simulink model "Modello_Irb1300_controllo_dinamico"  (R2024a)
settings: Solver=FixedStepAuto  StartTime=0.0  StopTime=16.0  FixedStep=0.05  RelTol=1e-3
values from neighbouring files (symbols this model uses):
  DH = [ ... (first row only)    [BackupRUN1.m]    (also in BackupRUN2.m; IRB1300_ABB6DOF_bodytree_mesh_RUN2.m)
undefined symbols (not defined in the file or in its folder): DiscIntNeverNeededParam, rb
libraries: vrlib x1
settings Model: Creator=giaki  LastModifiedBy=giaki
settings DataIOCC: SignalLogging=off

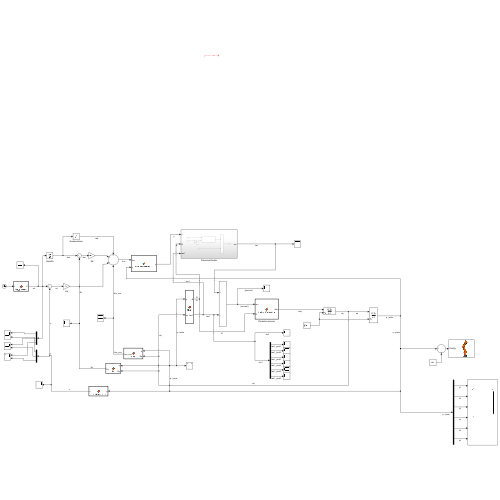
[thumbnail: Simulink's stored preview of the top-level diagram]
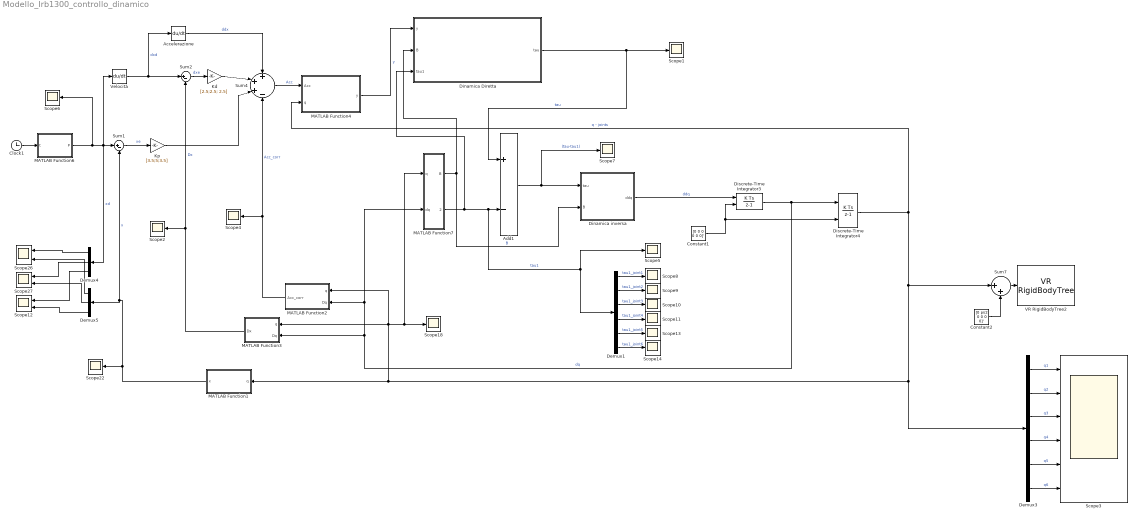
== system Modello_Irb1300_controllo_dinamico ==
  Accelerazione : Derivative
  Add1 : Sum  Inputs=+-
  Clock1 : Clock
  Constant1 : Constant  Value=[0 0 0 0 0 0]'
  Constant2 : Constant  Value=[0 pi/2 0 0 0 0]'
  Demux1 : Demux  Outputs=6
  Demux3 : Demux  Outputs=6
  Demux4 : Demux  Outputs=3
  Demux5 : Demux  Outputs=3
  Dinamica Diretta : Subsystem
  Dinamica inversa : MATLAB Function  TreatAsAtomicUnit=on
  Discrete-Time Integrator3 : DiscreteIntegrator  InitialConditionSource=external  SampleTime=-1  ICPrevOutput=DiscIntNeverNeededParam  ICPrevScaledInput=DiscIntNeverNeededParam
  Discrete-Time Integrator4 : DiscreteIntegrator  InitialConditionSource=external  SampleTime=-1  ICPrevOutput=DiscIntNeverNeededParam  ICPrevScaledInput=DiscIntNeverNeededParam
  Kd : Gain  Gain=[2.5;2.5; 2.5]
  Kp : Gain  Gain=[3.5;5;3.5]
  MATLAB Function1 : MATLAB Function  TreatAsAtomicUnit=on
  MATLAB Function2 : MATLAB Function  TreatAsAtomicUnit=on
  MATLAB Function3 : MATLAB Function  TreatAsAtomicUnit=on
  MATLAB Function4 : MATLAB Function  TreatAsAtomicUnit=on
  MATLAB Function6 : MATLAB Function  TreatAsAtomicUnit=on
  MATLAB Function7 : MATLAB Function  TreatAsAtomicUnit=on
  Scope{1..2,4..11,13..14,18,22} (14 alike) : Scope
  Scope12 : Scope  NumInputPorts=2
  Scope26 : Scope  NumInputPorts=2
  Scope27 : Scope  NumInputPorts=2
  Scope3 : Scope  NumInputPorts=6
  Sum1 : Sum  Inputs=|+-
  Sum2 : Sum  Inputs=|+-
  Sum4 : Sum  Inputs=+++-
  Sum7 : Sum  Inputs=|++
  VR RigidBodyTree2 : vrlib/VR RigidBodyTree  VrmlFile=robot_scene_2.x3d  RBT=Irb1300  useRBT=on  Ts=0.1  ForceViewerOpen=on
  Velocità : Derivative
  wires:
  ? -> ?
  MATLAB Function6/1(P) -> Scope6/1, Demux4/1, Sum1/1, Velocità/1  "xd"
  Demux4/2 -> Scope27/1
  Clock1/1 -> MATLAB Function6/1(t)
  Discrete-Time Integrator4/1 -> MATLAB Function1/1(q), MATLAB Function2/1(q), MATLAB Function3/1(q), Scope18/1, MATLAB Function7/1(q), Demux3/1, Sum7/1, MATLAB Function4/2(q)  "q - joints"
  MATLAB Function1/1(x) -> Sum1/2, Demux5/1, Scope22/1  "x"
  Sum2/1 -> Kd/1  "dxe"
  Demux4/3 -> Scope12/1
  MATLAB Function3/1(Dx) -> Scope2/1, Sum2/2  "Dx"
  Demux3/1 -> Scope3/1  "q1"
  Sum4/1 -> MATLAB Function4/1(Acc)  "Acc"
  Kd/1 -> Sum4/2
  Constant1/1 -> Discrete-Time Integrator3/2, Discrete-Time Integrator4/2
  Accelerazione/1 -> Sum4/1  "ddx"
  Demux5/1 -> Scope26/2
  Dinamica inversa/1(ddq) -> Discrete-Time Integrator3/1  "ddq"
  Demux3/3 -> Scope3/3  "q3"
  Add1/1 -> Scope7/1, Dinamica inversa/1(tau)  "(tau-tau1)"
  Discrete-Time Integrator3/1 -> MATLAB Function3/2(Dq), MATLAB Function7/2(dq), MATLAB Function2/2(Dq), Discrete-Time Integrator4/1  "dq"
  Sum1/1 -> Kp/1  "xe"
  Velocità/1 -> Sum2/1, Accelerazione/1  "dxd"
  MATLAB Function7/1(B) -> Dinamica Diretta/2(B), Dinamica inversa/2(B)  "B"
  Demux5/2 -> Scope27/2
  Dinamica Diretta/1(tau) -> Scope1/1, Add1/1  "tau"
  Demux3/5 -> Scope3/5  "q5"
  Sum7/1 -> VR RigidBodyTree2/1
  Demux4/1 -> Scope26/1
  Demux3/6 -> Scope3/6  "q6"
  Demux3/4 -> Scope3/4  "q4"
  Demux5/3 -> Scope12/2
  Constant2/1 -> Sum7/2
  MATLAB Function2/1(Acc_corr) -> Scope4/1, Sum4/4  "Acc_corr"
  MATLAB Function4/1(y) -> Dinamica Diretta/1(y)  "y"
  Demux3/2 -> Scope3/2  "q2"
  Kp/1 -> Sum4/3
  MATLAB Function7/2(tau1) -> Demux1/1, Scope5/1, Add1/2, Dinamica Diretta/3(tau1)  "tau1"
  Demux1/1 -> Scope8/1  "tau1_joint1"
  Demux1/2 -> Scope9/1  "tau1_joint2"
  Demux1/3 -> Scope10/1  "tau1_joint3"
  Demux1/4 -> Scope11/1  "tau1_joint4"
  Demux1/5 -> Scope13/1  "tau1_joint5"
  Demux1/6 -> Scope14/1  "tau1_joint6"

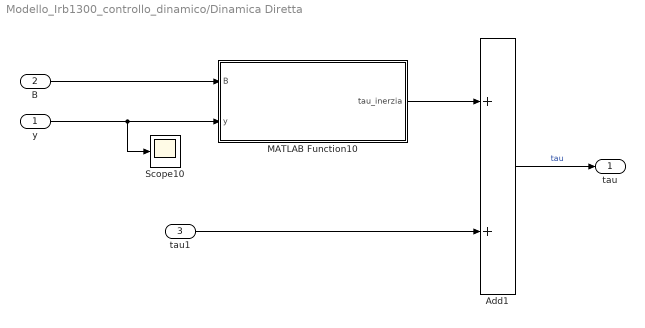
== system Modello_Irb1300_controllo_dinamico/Dinamica Diretta ==
  y : Inport
  B : Inport  Port=2
  tau1 : Inport  Port=3
  Add1 : Sum
  MATLAB Function10 : MATLAB Function  TreatAsAtomicUnit=on
  Scope10 : Scope
  tau : Outport
  wires:
  B/1 -> MATLAB Function10/1(B)
  MATLAB Function10/1(tau_inerzia) -> Add1/1
  y/1 -> Scope10/1, MATLAB Function10/2(y)
  Add1/1 -> tau/1  "tau"
  tau1/1 -> Add1/2

== matlab function Modello_Irb1300_controllo_dinamico/Dinamica Diretta/MATLAB Function10 ==
  data: B input size=[6,6]; tau_inerzia output; y input size=[6,1]
function tau_inerzia = calcolaTauInerzia(B,y)
    tau_inerzia = B*y;
end

== matlab function Modello_Irb1300_controllo_dinamico/MATLAB Function1 ==
  data: q input; x output
function x = directKinematics(q)

th1 = q(1);
th2 = q(2);
th3 = q(3);
th4 = q(4);
th5 = q(5);
th6 = q(6);

% T06

T = [
[  sin(th6)*(cos(th4)*sin(th1) + sin(th4)*(cos(th1)*sin(th3)*sin(th2 + pi/2) - cos(th1)*cos(th3)*cos(th2 + pi/2))) + cos(th6)*(cos(th5)*(sin(th1)*sin(th4) - cos(th4)*(cos(th1)*sin(th3)*sin(th2 + pi/2) - cos(th1)*cos(th3)*cos(th2 + pi/2))) - sin(th5)*(cos(th1)*cos(th3)*sin(th2 + pi/2) + cos(th1)*cos(th2 + pi/2)*sin(th3))), cos(th6)*(cos(th4)*sin(th1) + sin(th4)*(cos(th1)*sin(th3)*sin(th2 + pi/2) - cos(th1)*cos(th3)*cos(th2 + pi/2))) - sin(th6)*(cos(th5)*(sin(th1)*sin(th4) - cos(th4)*(cos(th1)*sin(th3)*sin(th2 + pi/2) - cos(th1)*cos(th3)*cos(th2 + pi/2))) - sin(th5)*(cos(th1)*cos(th3)*sin(th2 + pi/2) + cos(th1)*cos(th2 + pi/2)*sin(th3))), sin(th5)*(sin(th1)*sin(th4) - cos(th4)*(cos(th1)*sin(th3)*sin(th2 + pi/2) - cos(th1)*cos(th3)*cos(th2 + pi/2))) + cos(th5)*(cos(th1)*cos(th3)*sin(th2 + pi/2) + cos(th1)*cos(th2 + pi/2)*sin(th3)), cos(th1)/20 + (17*cos(th1)*cos(th2 + pi/2))/40 + (9*sin(th5)*(sin(th1)*sin(th4) - cos(th4)*(cos(th1)*sin(th3)*sin(th2 + pi/2) - cos(th1)*cos(th3)*cos(th2 + pi/2))))/50 + (9*cos(th5)*(cos(th1)*cos(th3)*sin(th2 + pi/2) + cos(th1)*cos(th2 + pi/2)*sin(th3)))/50 + (17*cos(th1)*cos(th3)*sin(th2 + pi/2))/40 + (17*cos(th1)*cos(th2 + pi/2)*sin(th3))/40 - (cos(th1)*sin(th3)*sin(th2 + pi/2))/25 + (cos(th1)*cos(th3)*cos(th2 + pi/2))/25]
[- sin(th6)*(cos(th1)*cos(th4) + sin(th4)*(cos(th3)*cos(th2 + pi/2)*sin(th1) - sin(th1)*sin(th3)*sin(th2 + pi/2))) - cos(th6)*(cos(th5)*(cos(th1)*sin(th4) - cos(th4)*(cos(th3)*cos(th2 + pi/2)*sin(th1) - sin(th1)*sin(th3)*sin(th2 + pi/2))) + sin(th5)*(cos(th3)*sin(th1)*sin(th2 + pi/2) + cos(th2 + pi/2)*sin(th1)*sin(th3))), sin(th6)*(cos(th5)*(cos(th1)*sin(th4) - cos(th4)*(cos(th3)*cos(th2 + pi/2)*sin(th1) - sin(th1)*sin(th3)*sin(th2 + pi/2))) + sin(th5)*(cos(th3)*sin(th1)*sin(th2 + pi/2) + cos(th2 + pi/2)*sin(th1)*sin(th3))) - cos(th6)*(cos(th1)*cos(th4) + sin(th4)*(cos(th3)*cos(th2 + pi/2)*sin(th1) - sin(th1)*sin(th3)*sin(th2 + pi/2))), cos(th5)*(cos(th3)*sin(th1)*sin(th2 + pi/2) + cos(th2 + pi/2)*sin(th1)*sin(th3)) - sin(th5)*(cos(th1)*sin(th4) - cos(th4)*(cos(th3)*cos(th2 + pi/2)*sin(th1) - sin(th1)*sin(th3)*sin(th2 + pi/2))), sin(th1)/20 + (17*cos(th2 + pi/2)*sin(th1))/40 - (9*sin(th5)*(cos(th1)*sin(th4) - cos(th4)*(cos(th3)*cos(th2 + pi/2)*sin(th1) - sin(th1)*sin(th3)*sin(th2 + pi/2))))/50 + (9*cos(th5)*(cos(th3)*sin(th1)*sin(th2 + pi/2) + cos(th2 + pi/2)*sin(th1)*sin(th3)))/50 + (cos(th3)*cos(th2 + pi/2)*sin(th1))/25 + (17*cos(th3)*sin(th1)*sin(th2 + pi/2))/40 + (17*cos(th2 + pi/2)*sin(th1)*sin(th3))/40 - (sin(th1)*sin(th3)*sin(th2 + pi/2))/25]
[                                                                                                    cos(th6)*(sin(th5)*(cos(th3)*cos(th2 + pi/2) - sin(th3)*sin(th2 + pi/2)) + cos(th4)*cos(th5)*(cos(th3)*sin(th2 + pi/2) + cos(th2 + pi/2)*sin(th3))) - sin(th4)*sin(th6)*(cos(th3)*sin(th2 + pi/2) + cos(th2 + pi/2)*sin(th3)),                                                                                                 - sin(th6)*(sin(th5)*(cos(th3)*cos(th2 + pi/2) - sin(th3)*sin(th2 + pi/2)) + cos(th4)*cos(th5)*(cos(th3)*sin(th2 + pi/2) + cos(th2 + pi/2)*sin(th3))) - cos(th6)*sin(th4)*(cos(th3)*sin(th2 + pi/2) + cos(th2 + pi/2)*sin(th3)),                                                           cos(th4)*sin(th5)*(cos(th3)*sin(th2 + pi/2) + cos(th2 + pi/2)*sin(th3)) - cos(th5)*(cos(th3)*cos(th2 + pi/2) - sin(th3)*sin(th2 + pi/2)),                                                                                                             (17*sin(th2 + pi/2))/40 - (17*cos(th3)*cos(th2 + pi/2))/40 + (cos(th3)*sin(th2 + pi/2))/25 + (cos(th2 + pi/2)*sin(th3))/25 + (17*sin(th3)*sin(th2 + pi/2))/40 - (9*cos(th5)*(cos(th3)*cos(th2 + pi/2) - sin(th3)*sin(th2 + pi/2)))/50 + (9*cos(th4)*sin(th5)*(cos(th3)*sin(th2 + pi/2) + cos(th2 + pi/2)*sin(th3)))/50 + 68/125]
[                                                                                                                                                                                                                                                                                                                                0,                                                                                                                                                                                                                                                                                                                               0,                                                                                                                                                                                                  0,                                                                                                                                                                                                                                                                                                                                                                                                                                           1]
 ];

x = T(1:3,4); % si estraggono i primi 3 valori della 4 colonna della T06 che rappresentano il vettore delle traslazioni 

end

== matlab function Modello_Irb1300_controllo_dinamico/MATLAB Function2 ==
  data: q input; Acc_corr output; Dq input
function Acc_corr = DJa(q,Dq)

th1 = q(1);
th2 = q(2);
th3 = q(3);
th4 = q(4);
th5 = q(5);
th6 = q(6);

% Velocità di giunto 
dth1 = Dq(1);
dth2 = Dq(2);
dth3 = Dq(3);
dth4 = Dq(4);
dth5 = Dq(5);
dth6 = Dq(6);


% Per il calcolo del DJ viene utilizzato lo script
% JacobianDerive_wrt_time.m 
% Viene utilizzato il DJ = DJp [3X1] di posizione


DJ = [
[(9*sin(th5)*(cos(th4)*(dth1*cos(th1)*sin(th3)*sin(th2 + pi/2) - dth1*cos(th1)*cos(th3)*cos(th2 + pi/2) + dth2*cos(th3)*sin(th1)*sin(th2 + pi/2) + dth2*cos(th2 + pi/2)*sin(th1)*sin(th3) + dth3*cos(th3)*sin(th1)*sin(th2 + pi/2) + dth3*cos(th2 + pi/2)*sin(th1)*sin(th3)) + dth4*sin(th4)*(cos(th3)*cos(th2 + pi/2)*sin(th1) - sin(th1)*sin(th3)*sin(th2 + pi/2)) + dth4*cos(th1)*cos(th4) - dth1*sin(th1)*sin(th4)))/50 - (9*cos(th5)*(dth1*cos(th1)*cos(th3)*sin(th2 + pi/2) + dth1*cos(th1)*cos(th2 + pi/2)*sin(th3) + dth2*cos(th3)*cos(th2 + pi/2)*sin(th1) + dth3*cos(th3)*cos(th2 + pi/2)*sin(th1) - dth2*sin(th1)*sin(th3)*sin(th2 + pi/2) - dth3*sin(th1)*sin(th3)*sin(th2 + pi/2)))/50 - (dth1*cos(th1))/20 + (9*dth5*sin(th5)*(cos(th3)*sin(th1)*sin(th2 + pi/2) + cos(th2 + pi/2)*sin(th1)*sin(th3)))/50 - (17*dth1*cos(th1)*cos(th2 + pi/2))/40 + (17*dth2*sin(th1)*sin(th2 + pi/2))/40 + (9*dth5*cos(th5)*(cos(th1)*sin(th4) - cos(th4)*(cos(th3)*cos(th2 + pi/2)*sin(th1) - sin(th1)*sin(th3)*sin(th2 + pi/2))))/50 - (dth1*cos(th1)*cos(th3)*cos(th2 + pi/2))/25 - (17*dth1*cos(th1)*cos(th3)*sin(th2 + pi/2))/40 - (17*dth1*cos(th1)*cos(th2 + pi/2)*sin(th3))/40 - (17*dth2*cos(th3)*cos(th2 + pi/2)*sin(th1))/40 - (17*dth3*cos(th3)*cos(th2 + pi/2)*sin(th1))/40 + (dth1*cos(th1)*sin(th3)*sin(th2 + pi/2))/25 + (dth2*cos(th3)*sin(th1)*sin(th2 + pi/2))/25 + (dth2*cos(th2 + pi/2)*sin(th1)*sin(th3))/25 + (dth3*cos(th3)*sin(th1)*sin(th2 + pi/2))/25 + (dth3*cos(th2 + pi/2)*sin(th1)*sin(th3))/25 + (17*dth2*sin(th1)*sin(th3)*sin(th2 + pi/2))/40 + (17*dth3*sin(th1)*sin(th3)*sin(th2 + pi/2))/40, (9*dth5*sin(th5)*(cos(th1)*sin(th3)*sin(th2 + pi/2) - cos(th1)*cos(th3)*cos(th2 + pi/2)))/50 - (9*cos(th5)*(dth1*cos(th3)*cos(th2 + pi/2)*sin(th1) + dth2*cos(th1)*cos(th3)*sin(th2 + pi/2) + dth2*cos(th1)*cos(th2 + pi/2)*sin(th3) + dth3*cos(th1)*cos(th3)*sin(th2 + pi/2) + dth3*cos(th1)*cos(th2 + pi/2)*sin(th3) - dth1*sin(th1)*sin(th3)*sin(th2 + pi/2)))/50 + (9*cos(th4)*sin(th5)*(dth1*cos(th3)*sin(th1)*sin(th2 + pi/2) - dth3*cos(th1)*cos(th3)*cos(th2 + pi/2) - dth2*cos(th1)*cos(th3)*cos(th2 + pi/2) + dth1*cos(th2 + pi/2)*sin(th1)*sin(th3) + dth2*cos(th1)*sin(th3)*sin(th2 + pi/2) + dth3*cos(th1)*sin(th3)*sin(th2 + pi/2)))/50 - (17*dth2*cos(th1)*cos(th2 + pi/2))/40 + (17*dth1*sin(th1)*sin(th2 + pi/2))/40 - (dth2*cos(th1)*cos(th3)*cos(th2 + pi/2))/25 - (dth3*cos(th1)*cos(th3)*cos(th2 + pi/2))/25 - (17*dth1*cos(th3)*cos(th2 + pi/2)*sin(th1))/40 - (17*dth2*cos(th1)*cos(th3)*sin(th2 + pi/2))/40 - (17*dth2*cos(th1)*cos(th2 + pi/2)*sin(th3))/40 - (17*dth3*cos(th1)*cos(th3)*sin(th2 + pi/2))/40 - (17*dth3*cos(th1)*cos(th2 + pi/2)*sin(th3))/40 + (dth1*cos(th3)*sin(th1)*sin(th2 + pi/2))/25 + (dth1*cos(th2 + pi/2)*sin(th1)*sin(th3))/25 + (dth2*cos(th1)*sin(th3)*sin(th2 + pi/2))/25 + (dth3*cos(th1)*sin(th3)*sin(th2 + pi/2))/25 + (17*dth1*sin(th1)*sin(th3)*sin(th2 + pi/2))/40 - (9*dth5*cos(th4)*cos(th5)*(cos(th1)*cos(th3)*sin(th2 + pi/2) + cos(th1)*cos(th2 + pi/2)*sin(th3)))/50 + (9*dth4*sin(th4)*sin(th5)*(cos(th1)*cos(th3)*sin(th2 + pi/2) + cos(th1)*cos(th2 + pi/2)*sin(th3)))/50, (9*dth5*sin(th5)*(cos(th1)*sin(th3)*sin(th2 + pi/2) - cos(th1)*cos(th3)*cos(th2 + pi/2)))/50 - (9*cos(th5)*(dth1*cos(th3)*cos(th2 + pi/2)*sin(th1) + dth2*cos(th1)*cos(th3)*sin(th2 + pi/2) + dth2*cos(th1)*cos(th2 + pi/2)*sin(th3) + dth3*cos(th1)*cos(th3)*sin(th2 + pi/2) + dth3*cos(th1)*cos(th2 + pi/2)*sin(th3) - dth1*sin(th1)*sin(th3)*sin(th2 + pi/2)))/50 + (9*cos(th4)*sin(th5)*(dth1*cos(th3)*sin(th1)*sin(th2 + pi/2) - dth3*cos(th1)*cos(th3)*cos(th2 + pi/2) - dth2*cos(th1)*cos(th3)*cos(th2 + pi/2) + dth1*cos(th2 + pi/2)*sin(th1)*sin(th3) + dth2*cos(th1)*sin(th3)*sin(th2 + pi/2) + dth3*cos(th1)*sin(th3)*sin(th2 + pi/2)))/50 - (dth2*cos(th1)*cos(th3)*cos(th2 + pi/2))/25 - (dth3*cos(th1)*cos(th3)*cos(th2 + pi/2))/25 - (17*dth1*cos(th3)*cos(th2 + pi/2)*sin(th1))/40 - (17*dth2*cos(th1)*cos(th3)*sin(th2 + pi/2))/40 - (17*dth2*cos(th1)*cos(th2 + pi/2)*sin(th3))/40 - (17*dth3*cos(th1)*cos(th3)*sin(th2 + pi/2))/40 - (17*dth3*cos(th1)*cos(th2 + pi/2)*sin(th3))/40 + (dth1*cos(th3)*sin(th1)*sin(th2 + pi/2))/25 + (dth1*cos(th2 + pi/2)*sin(th1)*sin(th3))/25 + (dth2*cos(th1)*sin(th3)*sin(th2 + pi/2))/25 + (dth3*cos(th1)*sin(th3)*sin(th2 + pi/2))/25 + (17*dth1*sin(th1)*sin(th3)*sin(th2 + pi/2))/40 - (9*dth5*cos(th4)*cos(th5)*(cos(th1)*cos(th3)*sin(th2 + pi/2) + cos(th1)*cos(th2 + pi/2)*sin(th3)))/50 + (9*dth4*sin(th4)*sin(th5)*(cos(th1)*cos(th3)*sin(th2 + pi/2) + cos(th1)*cos(th2 + pi/2)*sin(th3)))/50, (9*sin(th5)*(sin(th4)*(dth1*cos(th3)*cos(th2 + pi/2)*sin(th1) + dth2*cos(th1)*cos(th3)*sin(th2 + pi/2) + dth2*cos(th1)*cos(th2 + pi/2)*sin(th3) + dth3*cos(th1)*cos(th3)*sin(th2 + pi/2) + dth3*cos(th1)*cos(th2 + pi/2)*sin(th3) - dth1*sin(th1)*sin(th3)*sin(th2 + pi/2)) + dth4*cos(th4)*(cos(th1)*sin(th3)*sin(th2 + pi/2) - cos(th1)*cos(th3)*cos(th2 + pi/2)) + dth1*cos(th1)*cos(th4) - dth4*sin(th1)*sin(th4)))/50 + (9*dth5*cos(th5)*(cos(th4)*sin(th1) + sin(th4)*(cos(th1)*sin(th3)*sin(th2 + pi/2) - cos(th1)*cos(th3)*cos(th2 + pi/2))))/50, (9*sin(th5)*(dth1*cos(th3)*sin(th1)*sin(th2 + pi/2) - dth3*cos(th1)*cos(th3)*cos(th2 + pi/2) - dth2*cos(th1)*cos(th3)*cos(th2 + pi/2) + dth1*cos(th2 + pi/2)*sin(th1)*sin(th3) + dth2*cos(th1)*sin(th3)*sin(th2 + pi/2) + dth3*cos(th1)*sin(th3)*sin(th2 + pi/2)))/50 + (9*cos(th5)*(dth4*sin(th4)*(cos(th1)*sin(th3)*sin(th2 + pi/2) - cos(th1)*cos(th3)*cos(th2 + pi/2)) - cos(th4)*(dth1*cos(th3)*cos(th2 + pi/2)*sin(th1) + dth2*cos(th1)*cos(th3)*sin(th2 + pi/2) + dth2*cos(th1)*cos(th2 + pi/2)*sin(th3) + dth3*cos(th1)*cos(th3)*sin(th2 + pi/2) + dth3*cos(th1)*cos(th2 + pi/2)*sin(th3) - dth1*sin(th1)*sin(th3)*sin(th2 + pi/2)) + dth1*cos(th1)*sin(th4) + dth4*cos(th4)*sin(th1)))/50 - (9*dth5*cos(th5)*(cos(th1)*cos(th3)*sin(th2 + pi/2) + cos(th1)*cos(th2 + pi/2)*sin(th3)))/50 - (9*dth5*sin(th5)*(sin(th1)*sin(th4) - cos(th4)*(cos(th1)*sin(th3)*sin(th2 + pi/2) - cos(th1)*cos(th3)*cos(th2 + pi/2))))/50, 0]
[(9*sin(th5)*(dth4*sin(th4)*(cos(th1)*sin(th3)*sin(th2 + pi/2) - cos(th1)*cos(th3)*cos(th2 + pi/2)) - cos(th4)*(dth1*cos(th3)*cos(th2 + pi/2)*sin(th1) + dth2*cos(th1)*cos(th3)*sin(th2 + pi/2) + dth2*cos(th1)*cos(th2 + pi/2)*sin(th3) + dth3*cos(th1)*cos(th3)*sin(th2 + pi/2) + dth3*cos(th1)*cos(th2 + pi/2)*sin(th3) - dth1*sin(th1)*sin(th3)*sin(th2 + pi/2)) + dth1*cos(th1)*sin(th4) + dth4*cos(th4)*sin(th1)))/50 - (dth1*sin(th1))/20 - (9*cos(th5)*(dth1*cos(th3)*sin(th1)*sin(th2 + pi/2) - dth3*cos(th1)*cos(th3)*cos(th2 + pi/2) - dth2*cos(th1)*cos(th3)*cos(th2 + pi/2) + dth1*cos(th2 + pi/2)*sin(th1)*sin(th3) + dth2*cos(th1)*sin(th3)*sin(th2 + pi/2) + dth3*cos(th1)*sin(th3)*sin(th2 + pi/2)))/50 - (9*dth5*sin(th5)*(cos(th1)*cos(th3)*sin(th2 + pi/2) + cos(th1)*cos(th2 + pi/2)*sin(th3)))/50 - (17*dth1*cos(th2 + pi/2)*sin(th1))/40 - (17*dth2*cos(th1)*sin(th2 + pi/2))/40 + (9*dth5*cos(th5)*(sin(th1)*sin(th4) - cos(th4)*(cos(th1)*sin(th3)*sin(th2 + pi/2) - cos(th1)*cos(th3)*cos(th2 + pi/2))))/50 + (17*dth2*cos(th1)*cos(th3)*cos(th2 + pi/2))/40 + (17*dth3*cos(th1)*cos(th3)*cos(th2 + pi/2))/40 - (dth1*cos(th3)*cos(th2 + pi/2)*sin(th1))/25 - (dth2*cos(th1)*cos(th3)*sin(th2 + pi/2))/25 - (dth2*cos(th1)*cos(th2 + pi/2)*sin(th3))/25 - (dth3*cos(th1)*cos(th3)*sin(th2 + pi/2))/25 - (dth3*cos(th1)*cos(th2 + pi/2)*sin(th3))/25 - (17*dth1*cos(th3)*sin(th1)*sin(th2 + pi/2))/40 - (17*dth1*cos(th2 + pi/2)*sin(th1)*sin(th3))/40 - (17*dth2*cos(th1)*sin(th3)*sin(th2 + pi/2))/40 - (17*dth3*cos(th1)*sin(th3)*sin(th2 + pi/2))/40 + (dth1*sin(th1)*sin(th3)*sin(th2 + pi/2))/25, (9*dth4*sin(th4)*sin(th5)*(cos(th3)*sin(th1)*sin(th2 + pi/2) + cos(th2 + pi/2)*sin(th1)*sin(th3)))/50 - (9*dth5*sin(th5)*(cos(th3)*cos(th2 + pi/2)*sin(th1) - sin(th1)*sin(th3)*sin(th2 + pi/2)))/50 - (9*cos(th4)*sin(th5)*(dth1*cos(th1)*cos(th3)*sin(th2 + pi/2) + dth1*cos(th1)*cos(th2 + pi/2)*sin(th3) + dth2*cos(th3)*cos(th2 + pi/2)*sin(th1) + dth3*cos(th3)*cos(th2 + pi/2)*sin(th1) - dth2*sin(th1)*sin(th3)*sin(th2 + pi/2) - dth3*sin(th1)*sin(th3)*sin(th2 + pi/2)))/50 - (17*dth1*cos(th1)*sin(th2 + pi/2))/40 - (17*dth2*cos(th2 + pi/2)*sin(th1))/40 - (9*cos(th5)*(dth1*cos(th1)*sin(th3)*sin(th2 + pi/2) - dth1*cos(th1)*cos(th3)*cos(th2 + pi/2) + dth2*cos(th3)*sin(th1)*sin(th2 + pi/2) + dth2*cos(th2 + pi/2)*sin(th1)*sin(th3) + dth3*cos(th3)*sin(th1)*sin(th2 + pi/2) + dth3*cos(th2 + pi/2)*sin(th1)*sin(th3)))/50 + (17*dth1*cos(th1)*cos(th3)*cos(th2 + pi/2))/40 - (dth1*cos(th1)*cos(th3)*sin(th2 + pi/2))/25 - (dth1*cos(th1)*cos(th2 + pi/2)*sin(th3))/25 - (dth2*cos(th3)*cos(th2 + pi/2)*sin(th1))/25 - (dth3*cos(th3)*cos(th2 + pi/2)*sin(th1))/25 - (17*dth1*cos(th1)*sin(th3)*sin(th2 + pi/2))/40 - (17*dth2*cos(th3)*sin(th1)*sin(th2 + pi/2))/40 - (17*dth2*cos(th2 + pi/2)*sin(th1)*sin(th3))/40 - (17*dth3*cos(th3)*sin(th1)*sin(th2 + pi/2))/40 - (17*dth3*cos(th2 + pi/2)*sin(th1)*sin(th3))/40 + (dth2*sin(th1)*sin(th3)*sin(th2 + pi/2))/25 + (dth3*sin(th1)*sin(th3)*sin(th2 + pi/2))/25 - (9*dth5*cos(th4)*cos(th5)*(cos(th3)*sin(th1)*sin(th2 + pi/2) + cos(th2 + pi/2)*sin(th1)*sin(th3)))/50, (9*dth4*sin(th4)*sin(th5)*(cos(th3)*sin(th1)*sin(th2 + pi/2) + cos(th2 + pi/2)*sin(th1)*sin(th3)))/50 - (9*dth5*sin(th5)*(cos(th3)*cos(th2 + pi/2)*sin(th1) - sin(th1)*sin(th3)*sin(th2 + pi/2)))/50 - (9*cos(th4)*sin(th5)*(dth1*cos(th1)*cos(th3)*sin(th2 + pi/2) + dth1*cos(th1)*cos(th2 + pi/2)*sin(th3) + dth2*cos(th3)*cos(th2 + pi/2)*sin(th1) + dth3*cos(th3)*cos(th2 + pi/2)*sin(th1) - dth2*sin(th1)*sin(th3)*sin(th2 + pi/2) - dth3*sin(th1)*sin(th3)*sin(th2 + pi/2)))/50 - (9*cos(th5)*(dth1*cos(th1)*sin(th3)*sin(th2 + pi/2) - dth1*cos(th1)*cos(th3)*cos(th2 + pi/2) + dth2*cos(th3)*sin(th1)*sin(th2 + pi/2) + dth2*cos(th2 + pi/2)*sin(th1)*sin(th3) + dth3*cos(th3)*sin(th1)*sin(th2 + pi/2) + dth3*cos(th2 + pi/2)*sin(th1)*sin(th3)))/50 + (17*dth1*cos(th1)*cos(th3)*cos(th2 + pi/2))/40 - (dth1*cos(th1)*cos(th3)*sin(th2 + pi/2))/25 - (dth1*cos(th1)*cos(th2 + pi/2)*sin(th3))/25 - (dth2*cos(th3)*cos(th2 + pi/2)*sin(th1))/25 - (dth3*cos(th3)*cos(th2 + pi/2)*sin(th1))/25 - (17*dth1*cos(th1)*sin(th3)*sin(th2 + pi/2))/40 - (17*dth2*cos(th3)*sin(th1)*sin(th2 + pi/2))/40 - (17*dth2*cos(th2 + pi/2)*sin(th1)*sin(th3))/40 - (17*dth3*cos(th3)*sin(th1)*sin(th2 + pi/2))/40 - (17*dth3*cos(th2 + pi/2)*sin(th1)*sin(th3))/40 + (dth2*sin(th1)*sin(th3)*sin(th2 + pi/2))/25 + (dth3*sin(th1)*sin(th3)*sin(th2 + pi/2))/25 - (9*dth5*cos(th4)*cos(th5)*(cos(th3)*sin(th1)*sin(th2 + pi/2) + cos(th2 + pi/2)*sin(th1)*sin(th3)))/50, (9*sin(th5)*(sin(th4)*(dth1*cos(th1)*sin(th3)*sin(th2 + pi/2) - dth1*cos(th1)*cos(th3)*cos(th2 + pi/2) + dth2*cos(th3)*sin(th1)*sin(th2 + pi/2) + dth2*cos(th2 + pi/2)*sin(th1)*sin(th3) + dth3*cos(th3)*sin(th1)*sin(th2 + pi/2) + dth3*cos(th2 + pi/2)*sin(th1)*sin(th3)) - dth4*cos(th4)*(cos(th3)*cos(th2 + pi/2)*sin(th1) - sin(th1)*sin(th3)*sin(th2 + pi/2)) + dth1*cos(th4)*sin(th1) + dth4*cos(th1)*sin(th4)))/50 - (9*dth5*cos(th5)*(cos(th1)*cos(th4) + sin(th4)*(cos(th3)*cos(th2 + pi/2)*sin(th1) - sin(th1)*sin(th3)*sin(th2 + pi/2))))/50, (9*dth5*sin(th5)*(cos(th1)*sin(th4) - cos(th4)*(cos(th3)*cos(th2 + pi/2)*sin(th1) - sin(th1)*sin(th3)*sin(th2 + pi/2))))/50 - (9*sin(th5)*(dth1*cos(th1)*cos(th3)*sin(th2 + pi/2) + dth1*cos(th1)*cos(th2 + pi/2)*sin(th3) + dth2*cos(th3)*cos(th2 + pi/2)*sin(th1) + dth3*cos(th3)*cos(th2 + pi/2)*sin(th1) - dth2*sin(th1)*sin(th3)*sin(th2 + pi/2) - dth3*sin(th1)*sin(th3)*sin(th2 + pi/2)))/50 - (9*dth5*cos(th5)*(cos(th3)*sin(th1)*sin(th2 + pi/2) + cos(th2 + pi/2)*sin(th1)*sin(th3)))/50 - (9*cos(th5)*(cos(th4)*(dth1*cos(th1)*sin(th3)*sin(th2 + pi/2) - dth1*cos(th1)*cos(th3)*cos(th2 + pi/2) + dth2*cos(th3)*sin(th1)*sin(th2 + pi/2) + dth2*cos(th2 + pi/2)*sin(th1)*sin(th3) + dth3*cos(th3)*sin(th1)*sin(th2 + pi/2) + dth3*cos(th2 + pi/2)*sin(th1)*sin(th3)) + dth4*sin(th4)*(cos(th3)*cos(th2 + pi/2)*sin(th1) - sin(th1)*sin(th3)*sin(th2 + pi/2)) + dth4*cos(th1)*cos(th4) - dth1*sin(th1)*sin(th4)))/50, 0]
[                                                                                                                                                                                                                                                                                                                                                                                                                                                                                                                                                                                                                                                                                                                                                                                                                                                                                                                                                                                                                                                                                                                                                                                                                                                                                                                                                                                                                                                                                                                                                                                                                             0,                                                                                                                                                                                                                                                                                                                                                                                                                                                                                                                                                                                                                          (9*cos(th5)*(dth2*cos(th3)*cos(th2 + pi/2) + dth3*cos(th3)*cos(th2 + pi/2) - dth2*sin(th3)*sin(th2 + pi/2) - dth3*sin(th3)*sin(th2 + pi/2)))/50 - (17*dth2*sin(th2 + pi/2))/40 - (9*dth5*sin(th5)*(cos(th3)*sin(th2 + pi/2) + cos(th2 + pi/2)*sin(th3)))/50 + (17*dth2*cos(th3)*cos(th2 + pi/2))/40 + (17*dth3*cos(th3)*cos(th2 + pi/2))/40 - (dth2*cos(th3)*sin(th2 + pi/2))/25 - (dth2*cos(th2 + pi/2)*sin(th3))/25 - (dth3*cos(th3)*sin(th2 + pi/2))/25 - (dth3*cos(th2 + pi/2)*sin(th3))/25 - (17*dth2*sin(th3)*sin(th2 + pi/2))/40 - (17*dth3*sin(th3)*sin(th2 + pi/2))/40 - (9*cos(th4)*sin(th5)*(dth2*cos(th3)*sin(th2 + pi/2) + dth2*cos(th2 + pi/2)*sin(th3) + dth3*cos(th3)*sin(th2 + pi/2) + dth3*cos(th2 + pi/2)*sin(th3)))/50 + (9*dth5*cos(th4)*cos(th5)*(cos(th3)*cos(th2 + pi/2) - sin(th3)*sin(th2 + pi/2)))/50 - (9*dth4*sin(th4)*sin(th5)*(cos(th3)*cos(th2 + pi/2) - sin(th3)*sin(th2 + pi/2)))/50,                                                                                                                                                                                                                                                                                                                                                                                                                                                                                                                                                                         (9*cos(th5)*(dth2*cos(th3)*cos(th2 + pi/2) + dth3*cos(th3)*cos(th2 + pi/2) - dth2*sin(th3)*sin(th2 + pi/2) - dth3*sin(th3)*sin(th2 + pi/2)))/50 - (9*dth5*sin(th5)*(cos(th3)*sin(th2 + pi/2) + cos(th2 + pi/2)*sin(th3)))/50 + (17*dth2*cos(th3)*cos(th2 + pi/2))/40 + (17*dth3*cos(th3)*cos(th2 + pi/2))/40 - (dth2*cos(th3)*sin(th2 + pi/2))/25 - (dth2*cos(th2 + pi/2)*sin(th3))/25 - (dth3*cos(th3)*sin(th2 + pi/2))/25 - (dth3*cos(th2 + pi/2)*sin(th3))/25 - (17*dth2*sin(th3)*sin(th2 + pi/2))/40 - (17*dth3*sin(th3)*sin(th2 + pi/2))/40 - (9*cos(th4)*sin(th5)*(dth2*cos(th3)*sin(th2 + pi/2) + dth2*cos(th2 + pi/2)*sin(th3) + dth3*cos(th3)*sin(th2 + pi/2) + dth3*cos(th2 + pi/2)*sin(th3)))/50 + (9*dth5*cos(th4)*cos(th5)*(cos(th3)*cos(th2 + pi/2) - sin(th3)*sin(th2 + pi/2)))/50 - (9*dth4*sin(th4)*sin(th5)*(cos(th3)*cos(th2 + pi/2) - sin(th3)*sin(th2 + pi/2)))/50,                                                                                                                                                                                                                   - (9*sin(th4)*sin(th5)*(dth2*cos(th3)*cos(th2 + pi/2) + dth3*cos(th3)*cos(th2 + pi/2) - dth2*sin(th3)*sin(th2 + pi/2) - dth3*sin(th3)*sin(th2 + pi/2)))/50 - (9*dth4*cos(th4)*sin(th5)*(cos(th3)*sin(th2 + pi/2) + cos(th2 + pi/2)*sin(th3)))/50 - (9*dth5*cos(th5)*sin(th4)*(cos(th3)*sin(th2 + pi/2) + cos(th2 + pi/2)*sin(th3)))/50,                                                                                                                                                                                                                                                                                                                                                             (9*dth5*cos(th5)*(cos(th3)*cos(th2 + pi/2) - sin(th3)*sin(th2 + pi/2)))/50 - (9*sin(th5)*(dth2*cos(th3)*sin(th2 + pi/2) + dth2*cos(th2 + pi/2)*sin(th3) + dth3*cos(th3)*sin(th2 + pi/2) + dth3*cos(th2 + pi/2)*sin(th3)))/50 + (9*cos(th4)*cos(th5)*(dth2*cos(th3)*cos(th2 + pi/2) + dth3*cos(th3)*cos(th2 + pi/2) - dth2*sin(th3)*sin(th2 + pi/2) - dth3*sin(th3)*sin(th2 + pi/2)))/50 - (9*dth4*cos(th5)*sin(th4)*(cos(th3)*sin(th2 + pi/2) + cos(th2 + pi/2)*sin(th3)))/50 - (9*dth5*cos(th4)*sin(th5)*(cos(th3)*sin(th2 + pi/2) + cos(th2 + pi/2)*sin(th3)))/50, 0]
 ];

Acc_corr = DJ*Dq; 

end

== matlab function Modello_Irb1300_controllo_dinamico/MATLAB Function3 ==
  data: q input; Dx output size=[3,1]; Dq input
function Dx = Ja(q,Dq)
th1 = q(1);
th2 = q(2);
th3 = q(3);
th4 = q(4);
th5 = q(5);
th6 = q(6);

% Jacobiano di posizione J = Jp 
J = [
[(9*sin(th5)*(cos(th1)*sin(th4) - cos(th4)*(cos(th3)*cos(th2 + pi/2)*sin(th1) - sin(th1)*sin(th3)*sin(th2 + pi/2))))/50 - (17*cos(th2 + pi/2)*sin(th1))/40 - sin(th1)/20 - (9*cos(th5)*(cos(th3)*sin(th1)*sin(th2 + pi/2) + cos(th2 + pi/2)*sin(th1)*sin(th3)))/50 - (cos(th3)*cos(th2 + pi/2)*sin(th1))/25 - (17*cos(th3)*sin(th1)*sin(th2 + pi/2))/40 - (17*cos(th2 + pi/2)*sin(th1)*sin(th3))/40 + (sin(th1)*sin(th3)*sin(th2 + pi/2))/25, (17*cos(th1)*cos(th3)*cos(th2 + pi/2))/40 - (9*cos(th5)*(cos(th1)*sin(th3)*sin(th2 + pi/2) - cos(th1)*cos(th3)*cos(th2 + pi/2)))/50 - (cos(th1)*cos(th3)*sin(th2 + pi/2))/25 - (cos(th1)*cos(th2 + pi/2)*sin(th3))/25 - (17*cos(th1)*sin(th3)*sin(th2 + pi/2))/40 - (9*cos(th4)*sin(th5)*(cos(th1)*cos(th3)*sin(th2 + pi/2) + cos(th1)*cos(th2 + pi/2)*sin(th3)))/50 - (17*cos(th1)*sin(th2 + pi/2))/40, (17*cos(th1)*cos(th3)*cos(th2 + pi/2))/40 - (cos(th1)*cos(th3)*sin(th2 + pi/2))/25 - (cos(th1)*cos(th2 + pi/2)*sin(th3))/25 - (17*cos(th1)*sin(th3)*sin(th2 + pi/2))/40 - (9*cos(th4)*sin(th5)*(cos(th1)*cos(th3)*sin(th2 + pi/2) + cos(th1)*cos(th2 + pi/2)*sin(th3)))/50 - (9*cos(th5)*(cos(th1)*sin(th3)*sin(th2 + pi/2) - cos(th1)*cos(th3)*cos(th2 + pi/2)))/50,  (9*sin(th5)*(cos(th4)*sin(th1) + sin(th4)*(cos(th1)*sin(th3)*sin(th2 + pi/2) - cos(th1)*cos(th3)*cos(th2 + pi/2))))/50,   (9*cos(th5)*(sin(th1)*sin(th4) - cos(th4)*(cos(th1)*sin(th3)*sin(th2 + pi/2) - cos(th1)*cos(th3)*cos(th2 + pi/2))))/50 - (9*sin(th5)*(cos(th1)*cos(th3)*sin(th2 + pi/2) + cos(th1)*cos(th2 + pi/2)*sin(th3)))/50, 0]
[cos(th1)/20 + (17*cos(th1)*cos(th2 + pi/2))/40 + (9*sin(th5)*(sin(th1)*sin(th4) - cos(th4)*(cos(th1)*sin(th3)*sin(th2 + pi/2) - cos(th1)*cos(th3)*cos(th2 + pi/2))))/50 + (9*cos(th5)*(cos(th1)*cos(th3)*sin(th2 + pi/2) + cos(th1)*cos(th2 + pi/2)*sin(th3)))/50 + (17*cos(th1)*cos(th3)*sin(th2 + pi/2))/40 + (17*cos(th1)*cos(th2 + pi/2)*sin(th3))/40 - (cos(th1)*sin(th3)*sin(th2 + pi/2))/25 + (cos(th1)*cos(th3)*cos(th2 + pi/2))/25, (9*cos(th5)*(cos(th3)*cos(th2 + pi/2)*sin(th1) - sin(th1)*sin(th3)*sin(th2 + pi/2)))/50 - (17*sin(th1)*sin(th2 + pi/2))/40 + (17*cos(th3)*cos(th2 + pi/2)*sin(th1))/40 - (cos(th3)*sin(th1)*sin(th2 + pi/2))/25 - (cos(th2 + pi/2)*sin(th1)*sin(th3))/25 - (17*sin(th1)*sin(th3)*sin(th2 + pi/2))/40 - (9*cos(th4)*sin(th5)*(cos(th3)*sin(th1)*sin(th2 + pi/2) + cos(th2 + pi/2)*sin(th1)*sin(th3)))/50, (9*cos(th5)*(cos(th3)*cos(th2 + pi/2)*sin(th1) - sin(th1)*sin(th3)*sin(th2 + pi/2)))/50 + (17*cos(th3)*cos(th2 + pi/2)*sin(th1))/40 - (cos(th3)*sin(th1)*sin(th2 + pi/2))/25 - (cos(th2 + pi/2)*sin(th1)*sin(th3))/25 - (17*sin(th1)*sin(th3)*sin(th2 + pi/2))/40 - (9*cos(th4)*sin(th5)*(cos(th3)*sin(th1)*sin(th2 + pi/2) + cos(th2 + pi/2)*sin(th1)*sin(th3)))/50, -(9*sin(th5)*(cos(th1)*cos(th4) + sin(th4)*(cos(th3)*cos(th2 + pi/2)*sin(th1) - sin(th1)*sin(th3)*sin(th2 + pi/2))))/50, - (9*cos(th5)*(cos(th1)*sin(th4) - cos(th4)*(cos(th3)*cos(th2 + pi/2)*sin(th1) - sin(th1)*sin(th3)*sin(th2 + pi/2))))/50 - (9*sin(th5)*(cos(th3)*sin(th1)*sin(th2 + pi/2) + cos(th2 + pi/2)*sin(th1)*sin(th3)))/50, 0]
[                                                                                                                                                                                                                                                                                                                                                                                                                                          0,                                                                                  (17*cos(th2 + pi/2))/40 + (cos(th3)*cos(th2 + pi/2))/25 + (17*cos(th3)*sin(th2 + pi/2))/40 + (17*cos(th2 + pi/2)*sin(th3))/40 - (sin(th3)*sin(th2 + pi/2))/25 + (9*cos(th5)*(cos(th3)*sin(th2 + pi/2) + cos(th2 + pi/2)*sin(th3)))/50 + (9*cos(th4)*sin(th5)*(cos(th3)*cos(th2 + pi/2) - sin(th3)*sin(th2 + pi/2)))/50,                                                                         (cos(th3)*cos(th2 + pi/2))/25 + (17*cos(th3)*sin(th2 + pi/2))/40 + (17*cos(th2 + pi/2)*sin(th3))/40 - (sin(th3)*sin(th2 + pi/2))/25 + (9*cos(th5)*(cos(th3)*sin(th2 + pi/2) + cos(th2 + pi/2)*sin(th3)))/50 + (9*cos(th4)*sin(th5)*(cos(th3)*cos(th2 + pi/2) - sin(th3)*sin(th2 + pi/2)))/50,                                         -(9*sin(th4)*sin(th5)*(cos(th3)*sin(th2 + pi/2) + cos(th2 + pi/2)*sin(th3)))/50,                                                             (9*sin(th5)*(cos(th3)*cos(th2 + pi/2) - sin(th3)*sin(th2 + pi/2)))/50 + (9*cos(th4)*cos(th5)*(cos(th3)*sin(th2 + pi/2) + cos(th2 + pi/2)*sin(th3)))/50, 0]
];

Dx = J*Dq;

end

== matlab function Modello_Irb1300_controllo_dinamico/MATLAB Function4 ==
  data: Acc input; y output size=[6,1]; q input
function y = inverseKinematic(Acc,q)

th1 = q(1);
th2 = q(2);
th3 = q(3);
th4 = q(4);
th5 = q(5);
th6 = q(6);

%Jacobiano valutato nel tempo sul vettore q  
J = [
[(9*sin(th5)*(cos(th1)*sin(th4) - cos(th4)*(cos(th3)*cos(th2 + pi/2)*sin(th1) - sin(th1)*sin(th3)*sin(th2 + pi/2))))/50 - (17*cos(th2 + pi/2)*sin(th1))/40 - sin(th1)/20 - (9*cos(th5)*(cos(th3)*sin(th1)*sin(th2 + pi/2) + cos(th2 + pi/2)*sin(th1)*sin(th3)))/50 - (cos(th3)*cos(th2 + pi/2)*sin(th1))/25 - (17*cos(th3)*sin(th1)*sin(th2 + pi/2))/40 - (17*cos(th2 + pi/2)*sin(th1)*sin(th3))/40 + (sin(th1)*sin(th3)*sin(th2 + pi/2))/25, (17*cos(th1)*cos(th3)*cos(th2 + pi/2))/40 - (9*cos(th5)*(cos(th1)*sin(th3)*sin(th2 + pi/2) - cos(th1)*cos(th3)*cos(th2 + pi/2)))/50 - (cos(th1)*cos(th3)*sin(th2 + pi/2))/25 - (cos(th1)*cos(th2 + pi/2)*sin(th3))/25 - (17*cos(th1)*sin(th3)*sin(th2 + pi/2))/40 - (9*cos(th4)*sin(th5)*(cos(th1)*cos(th3)*sin(th2 + pi/2) + cos(th1)*cos(th2 + pi/2)*sin(th3)))/50 - (17*cos(th1)*sin(th2 + pi/2))/40, (17*cos(th1)*cos(th3)*cos(th2 + pi/2))/40 - (cos(th1)*cos(th3)*sin(th2 + pi/2))/25 - (cos(th1)*cos(th2 + pi/2)*sin(th3))/25 - (17*cos(th1)*sin(th3)*sin(th2 + pi/2))/40 - (9*cos(th4)*sin(th5)*(cos(th1)*cos(th3)*sin(th2 + pi/2) + cos(th1)*cos(th2 + pi/2)*sin(th3)))/50 - (9*cos(th5)*(cos(th1)*sin(th3)*sin(th2 + pi/2) - cos(th1)*cos(th3)*cos(th2 + pi/2)))/50,  (9*sin(th5)*(cos(th4)*sin(th1) + sin(th4)*(cos(th1)*sin(th3)*sin(th2 + pi/2) - cos(th1)*cos(th3)*cos(th2 + pi/2))))/50,   (9*cos(th5)*(sin(th1)*sin(th4) - cos(th4)*(cos(th1)*sin(th3)*sin(th2 + pi/2) - cos(th1)*cos(th3)*cos(th2 + pi/2))))/50 - (9*sin(th5)*(cos(th1)*cos(th3)*sin(th2 + pi/2) + cos(th1)*cos(th2 + pi/2)*sin(th3)))/50, 0]
[cos(th1)/20 + (17*cos(th1)*cos(th2 + pi/2))/40 + (9*sin(th5)*(sin(th1)*sin(th4) - cos(th4)*(cos(th1)*sin(th3)*sin(th2 + pi/2) - cos(th1)*cos(th3)*cos(th2 + pi/2))))/50 + (9*cos(th5)*(cos(th1)*cos(th3)*sin(th2 + pi/2) + cos(th1)*cos(th2 + pi/2)*sin(th3)))/50 + (17*cos(th1)*cos(th3)*sin(th2 + pi/2))/40 + (17*cos(th1)*cos(th2 + pi/2)*sin(th3))/40 - (cos(th1)*sin(th3)*sin(th2 + pi/2))/25 + (cos(th1)*cos(th3)*cos(th2 + pi/2))/25, (9*cos(th5)*(cos(th3)*cos(th2 + pi/2)*sin(th1) - sin(th1)*sin(th3)*sin(th2 + pi/2)))/50 - (17*sin(th1)*sin(th2 + pi/2))/40 + (17*cos(th3)*cos(th2 + pi/2)*sin(th1))/40 - (cos(th3)*sin(th1)*sin(th2 + pi/2))/25 - (cos(th2 + pi/2)*sin(th1)*sin(th3))/25 - (17*sin(th1)*sin(th3)*sin(th2 + pi/2))/40 - (9*cos(th4)*sin(th5)*(cos(th3)*sin(th1)*sin(th2 + pi/2) + cos(th2 + pi/2)*sin(th1)*sin(th3)))/50, (9*cos(th5)*(cos(th3)*cos(th2 + pi/2)*sin(th1) - sin(th1)*sin(th3)*sin(th2 + pi/2)))/50 + (17*cos(th3)*cos(th2 + pi/2)*sin(th1))/40 - (cos(th3)*sin(th1)*sin(th2 + pi/2))/25 - (cos(th2 + pi/2)*sin(th1)*sin(th3))/25 - (17*sin(th1)*sin(th3)*sin(th2 + pi/2))/40 - (9*cos(th4)*sin(th5)*(cos(th3)*sin(th1)*sin(th2 + pi/2) + cos(th2 + pi/2)*sin(th1)*sin(th3)))/50, -(9*sin(th5)*(cos(th1)*cos(th4) + sin(th4)*(cos(th3)*cos(th2 + pi/2)*sin(th1) - sin(th1)*sin(th3)*sin(th2 + pi/2))))/50, - (9*cos(th5)*(cos(th1)*sin(th4) - cos(th4)*(cos(th3)*cos(th2 + pi/2)*sin(th1) - sin(th1)*sin(th3)*sin(th2 + pi/2))))/50 - (9*sin(th5)*(cos(th3)*sin(th1)*sin(th2 + pi/2) + cos(th2 + pi/2)*sin(th1)*sin(th3)))/50, 0]
[                                                                                                                                                                                                                                                                                                                                                                                                                                          0,                                                                                  (17*cos(th2 + pi/2))/40 + (cos(th3)*cos(th2 + pi/2))/25 + (17*cos(th3)*sin(th2 + pi/2))/40 + (17*cos(th2 + pi/2)*sin(th3))/40 - (sin(th3)*sin(th2 + pi/2))/25 + (9*cos(th5)*(cos(th3)*sin(th2 + pi/2) + cos(th2 + pi/2)*sin(th3)))/50 + (9*cos(th4)*sin(th5)*(cos(th3)*cos(th2 + pi/2) - sin(th3)*sin(th2 + pi/2)))/50,                                                                         (cos(th3)*cos(th2 + pi/2))/25 + (17*cos(th3)*sin(th2 + pi/2))/40 + (17*cos(th2 + pi/2)*sin(th3))/40 - (sin(th3)*sin(th2 + pi/2))/25 + (9*cos(th5)*(cos(th3)*sin(th2 + pi/2) + cos(th2 + pi/2)*sin(th3)))/50 + (9*cos(th4)*sin(th5)*(cos(th3)*cos(th2 + pi/2) - sin(th3)*sin(th2 + pi/2)))/50,                                         -(9*sin(th4)*sin(th5)*(cos(th3)*sin(th2 + pi/2) + cos(th2 + pi/2)*sin(th3)))/50,                                                             (9*sin(th5)*(cos(th3)*cos(th2 + pi/2) - sin(th3)*sin(th2 + pi/2)))/50 + (9*cos(th4)*cos(th5)*(cos(th3)*sin(th2 + pi/2) + cos(th2 + pi/2)*sin(th3)))/50, 0] 
];

Jinv = pinv (J); % Inverte il Jacobiano 
y = Jinv*Acc;    % Moltiplica il Jacobiano inverso per il vettore delle accelerazioni Acc 
pause (0.01);

end

== matlab function Modello_Irb1300_controllo_dinamico/Dinamica inversa ==
  data: tau input size=[6,1]; ddq output; B input
% Dinamica inversa
function ddq = IndirectDynamics(tau, B)
    Binv = pinv(B); % Calcola la pseudo-inversa di B
    ddq = Binv*tau; % Calcola le accelerazioni di giunto 
end

== matlab function Modello_Irb1300_controllo_dinamico/MATLAB Function6 ==
  data: t input; P output
function P = traj_planner(t)
% Intervallo di tempo
ti = 0;
tf = 16;
% Traslazione temporale 
t = t - ti;
tf = tf - ti;

% Posizioni nello spazio cartesiano riferito al frame di base del robot
Pi = [0.65 0 1.009].';      % [3x1] (m) Posizione dell'end-effector iniziale  
Pf = [0.65 0 1.009].';     % [3x1] (m) Posizione dell'end-effector finale 
%Pf = [-0.374 -0.4 0.63].';  % [3x1] (m) Pf = Pi per l'analisi statica
delta_P = Pf - Pi;

% Incremento dell'accelerazione del 10% per garantire 
% che sia superiore al valore nominale

Acc=(4* delta_P/(tf^2)) * 1.10;

% Tempi di intervallo delle rampe di accelerazione 
tc1= tf/2 - sqrt(tf^2/4 - norm(delta_P)/norm(Acc));
tc2 = tf/2 + sqrt(tf^2/4 - norm(delta_P)/norm(Acc));

% Traiettoria
P = Pi;

if t >= 0 && t < tc1
    P = Pi + 1/2 * Acc * t^2;
elseif t >= tc1 && t < tc2
    P = Pi + Acc* tc1* (t - tc1/2);
elseif t >= tc2 && t < tf
    P = Pf - 1/2 * Acc * (tf - t)^2;
elseif t >= tf
    P = Pf;
end

end

== matlab function Modello_Irb1300_controllo_dinamico/MATLAB Function7 ==
  data: q input size=[6,1]; B output size=[6,6]; dq input size=[6,1]; tau1 output size=[6,1]; rb parameter Bus: slBus1; DH parameter
function [B, tau1] = RNE(q,dq,rb, DH)

n = length (q);    % Numero di giunti
B = zeros (n,n);   % Inizializzazione della matrice delle masse
I = eye (n);       % Inizializzazione della matrice Identità 
g = [0; 0; -9.81]; % Inizializzazione dell'array dell'accelerazioni [m/s^2]

for i=1:n
B(:,i) = RNE_Calc(q,zeros(n,1), I(:,i), rb, DH,g);
%B(:,i) = RNE_Calc(q,zeros(n,1), I(:,i), rb, DH); % Gravità = 0 [m/s^2]
end

tau1 = RNE_Calc(q, dq, zeros(n,1), rb,DH,g);
%tau1 = RNE_Calc(q, dq, zeros(n,1), rb, DH);      % Gravità = 0 [m/s^2]

end
